simulink model "mouse"  (R2024b)
settings: Solver=VariableStepAuto  StartTime=0.0  StopTime=inf  RelTol=1e-3
settings Model: Creator=kev  LastModifiedBy=kev

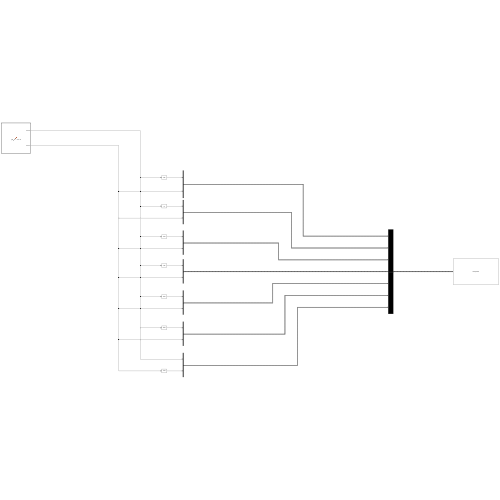
[thumbnail: Simulink's stored preview of the top-level diagram]
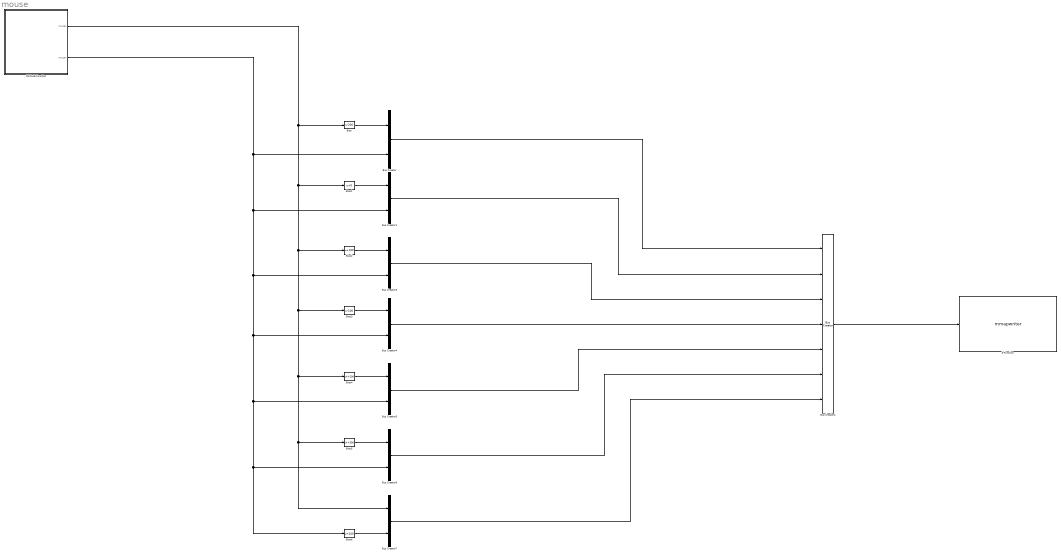
== system mouse ==
  Bias : Bias  Bias=-200  SaturateOnIntegerOverflow=off
  Bias1 : Bias  SaturateOnIntegerOverflow=off
  Bias2 : Bias  Bias=100  SaturateOnIntegerOverflow=off
  Bias3 : Bias  Bias=-100  SaturateOnIntegerOverflow=off
  Bias4 : Bias  Bias=+200  SaturateOnIntegerOverflow=off
  Bias5 : Bias  Bias=+300  SaturateOnIntegerOverflow=off
  Bias6 : Bias  Bias=100  SaturateOnIntegerOverflow=off
  Bus Creator{,1,3..7} (7 alike) : BusCreator  Inputs=2  OutDataTypeStr=Bus: MouseBus  NonVirtualBus=on
      settings: InheritFromInputs=off
  Bus Creator2 : BusCreator  Inputs=7  OutDataTypeStr=Bus: FullBus  NonVirtualBus=on
      settings: InheritFromInputs=off
  MATLAB Function : MATLAB Function  TreatAsAtomicUnit=on
  S-Function : S-Function  FunctionName=mmapwriter  Parameters=FullBus, 'Testing'  SFunctionDeploymentMode=off  EnableBusSupport=off
  wires:
  Bias/1 -> Bus Creator/1
  Bias1/1 -> Bus Creator1/1
  Bus Creator/1 -> Bus Creator2/1
  Bus Creator2/1 -> S-Function/1
  Bus Creator1/1 -> Bus Creator2/2
  Bias2/1 -> Bus Creator3/1
  Bias3/1 -> Bus Creator4/1
  Bus Creator4/1 -> Bus Creator2/4
  Bias4/1 -> Bus Creator5/1
  Bias5/1 -> Bus Creator6/1
  Bus Creator6/1 -> Bus Creator2/6
  Bus Creator7/1 -> Bus Creator2/7
  MATLAB Function/2(mouseY) -> Bias6/1, Bus Creator6/2, Bus Creator5/2, Bus Creator4/2, Bus Creator3/2, Bus Creator1/2, Bus Creator/2
  MATLAB Function/1(mouseX) -> Bus Creator7/1, Bias5/1, Bias4/1, Bias3/1, Bias2/1, Bias1/1, Bias/1
  Bias6/1 -> Bus Creator7/2
  Bus Creator3/1 -> Bus Creator2/3
  Bus Creator5/1 -> Bus Creator2/5

== matlab function mouse/MATLAB Function ==
  data: mouseX output; mouseY output
function [mouseX, mouseY] = get_mouse_info()
    coder.extrinsic('GetMouse');
    screen_nr = 0;
    mouse_nr = 0;

    mouseX = double(0);
    mouseY = double(0);
    
    [mouseX, mouseY] = GetMouse(screen_nr, mouse_nr);   

end
